simulink model "sf_newtons_cradle"  (R2017b)
settings: Solver=ode45  StartTime=0.0  StopTime=5  RelTol=1e-3
settings Model: Creator=The MathWorks, Inc.  LastModifiedBy=The MathWorks, Inc.
settings DataIOCC: LimitDataPoints=on  SaveFormat=Array
settings OptimizationCC: BlockReduction=off  BooleanDataType=off  ExpressionDepthLimit=2147483647  InitFltsAndDblsToZero=on  LifeSpan=inf
settings DebuggingCC: UnderspecifiedInitializationDetection=Classic  MergeDetectMultiDrivingBlocksExec=none  SignalResolutionControl=TryResolveAllWithWarning  FcnCallInpInsideContextMsg=warning  StateNameClashWarn=warning  StrictBusMsg=Warning  SFUnexpectedBacktrackingDiag=warning  SFNoUnconditionalDefaultTransitionDiag=warning  SFExecutionAtInitializationDiag=none
settings HardwareCC: ProdBitPerPointer=32  ProdBitPerSizeT=32  ProdBitPerPtrDiffT=32  ProdLargestAtomicFloat=None  ProdIntDivRoundTo=Undefined  ProdEndianess=Unspecified  ProdWordSize=32  ProdHWDeviceType=32-bit Generic  TargetUnknown=on
settings ModelReferenceCC: PropagateSignalLabelsOutOfModel=off
settings SFSimCC: SFSimEcho=off  SimParseCustomCode=off
settings CodeAppCC: StateflowObjectComments=on
settings GRTTargetCC: TargetFcnLib=ansi_tfl_tmw_new.mat  TargetLangStandard=C89/C90 (ANSI)  GeneratePreprocessorConditionals=Disable all  CombineOutputUpdateFcns=off  GRTInterface=on
settings ConfigComp: CovMetricSettings=dw  CovHtmlReporting=on  CovSaveCumulativeToWorkspaceVar=on  CovSaveSingleToWorkspaceVar=on  CovExternalEMLEnable=off  CovSFcnEnable=off

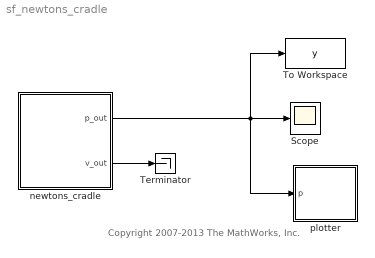
== system sf_newtons_cradle ==
  note: Copyright 2007-2013 The MathWorks, Inc.
  Scope : Scope
  Terminator : Terminator
  To Workspace : ToWorkspace  VariableName=y  SampleTime=-1
  newtons_cradle : Stateflow chart  TreatAsAtomicUnit=on
  plotter : Stateflow chart  TreatAsAtomicUnit=on
  wires:
  newtons_cradle/1(p_out) -> Scope/1, To Workspace/1, plotter/1(p)
  newtons_cradle/2(v_out) -> Terminator/1

== stateflow chart sf_newtons_cradle/newtons_cradle ==
  settings: updateMethod=CONTINUOUS  executeAtInitialization=1  initializeOutput=1
  state FreeDynamics
    du:
    p_out = p;
    v_out = v;
    p_dot = v;
    v_dot = -g/l*sin(p);
  state resetPositionsAndVelocities [function]
    (default) -> (junction 22) : {i=0;}
    (junction 22) -> (junction 24) [order 1] : [i < k-1]
    (junction 17) -> (junction 22) : {i++;}
    (junction 24) -> (junction 17) [order 2]
    (junction 24) -> (junction 17) [order 1] : [p[i] < p[i+1]]
        | {
        | // swap positions
        | tmp = p[i];
        | p[i] = p[i+1];
        | p[i+1] = tmp;
        | // swap velocities
        | tmp = v[i];
        | v[i] = v[i+1];
        | v[i+1] = tmp;
        | }
    (junction 22) -> (junction 23) [order 2]
  state collision = isCollisionPossible [function]
    (default) -> (junction 18) : {i=0;}
    (junction 18) -> (junction 20) [order 1] : [i < k-1]
    (junction 20) -> (junction 18) [order 2] : {i++;}
    (junction 18) -> (junction 19) [order 2] : {
        | collision = 0;
        | }
    (junction 20) -> (junction 21) [order 1] : [p[i] < p[i+1]]
        | {
        | collision = 1;
        | }
  (default) -> FreeDynamics : {
      | p = 0;
      | v = 0;
      | p[0] = pi/6;
      | p[1] = pi/6;
      |
      | // uncomment the lines below to see
      | // some interesting behavior
      | // p[k-3] = -pi/6;
      | // p[k-2] = -pi/6;
      | // p[k-1] = -pi/6;
      | // v[0] = 2;
      | }
  FreeDynamics -> FreeDynamics : [isCollisionPossible()]
      | { resetPositionsAndVelocities(); }
  data: i temporary double; tmp temporary double; collision function_output double; i temporary double; p_out output double size=k; v_out output double size=k; g constant double =9.81; l constant double =1; pi constant double =3.141; p local double size=k; v local double size=k; k constant int32 =7
  data p settings: updateMethod=SF_CONTINUOUS_TIME_DATA
  data v settings: updateMethod=SF_CONTINUOUS_TIME_DATA

== stateflow chart sf_newtons_cradle/plotter ==
  settings: updateMethod=DISCRETE  sampleTime=0.1
  state A
    du:
    ml.sf_newtons_cradle_plotter(p);
  data: p input double
